simulink model "soundTest"  (R2019a)
settings: Solver=VariableStepAuto  StartTime=0.0  StopTime=inf  RelTol=1e-3
libraries: dspsnks4 x1, dspvision x1
settings Model: Creator=CIT_007  LastModifiedBy=CIT_007

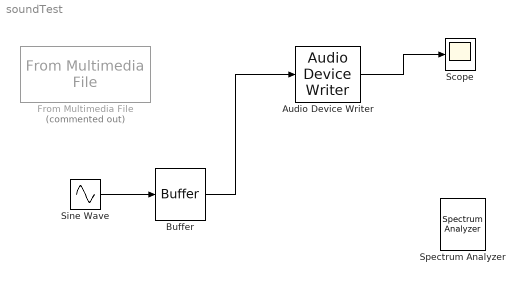
== system soundTest ==
  Audio Device Writer : dspsnks4/Audio Device Writer  Driver=DirectSound  Device=Default  InheritSampleRate=on  SampleRate=44100  BitDepth=16-bit integer  BufferSize=4096  NumBuffers=10  DefaultOutputChannelMapping=off  OutputChannelMapping=1:1  OutputNumUnderrunSamples=on  DriverIdx=1  DeviceWarnFlag=''
  Buffer : Buffer  N=1024  OutputFrames=off
  From Multimedia File : dspvision/From Multimedia File  Commented=on  inputFilename=speech_dft.mp3  readRange=[1 Inf]  loop=on  numPlays=inf  outputStreams=Audio only  videoDataType=single  audioDataType=double  inheritSampleTime=on  userDefinedSampleTime=1/30  noAudioOutput=off  isIntensityVideo=off  fourcc=RGB  colorVideoFormat=Separate color signals  outputEOF=off  dataOrg=Column-major  audioFrameSize=1024  computeAudioFrameSize=off  outSamplingMode=Sample based
      settings: SourceProductName=DSP System Toolbox  SourceProductBaseCode=DS
  Scope : Scope
  Sine Wave : Sin  Frequency=2*pi*1000  SampleTime=1/44100
  Spectrum Analyzer : SpectrumAnalyzer
  wires:
  Audio Device Writer/1 -> Scope/1
  Sine Wave/1 -> Buffer/1
  Buffer/1 -> Audio Device Writer/1
